simulink model "testUDPReceiveRoute"  (R2024a)
settings: Solver=FixedStepAuto  StartTime=0.0  StopTime=inf  FixedStep=1e-3  RelTol=1e-3
model workspace (MAT data in the model file):
  teste = Simulink.Parameter
  teste.Value = "Variable1"
  teste.Complexity = 'real'
  teste.Dimensions = [1 1]
  teste.DataType = 'string'
  teste1 = Simulink.Parameter
  teste1.Value = 1
  teste1.Complexity = 'real'
  teste1.Dimensions = [1 1]
  teste1.DataType = 'auto'
libraries: slrealtimeutilitieslib x1, slrealtimetgmanagement x1, slrealtimeiplib x1
settings Model: Creator=matlab.cut  LastModifiedBy=matlab.cut
settings SolverCC: ConcurrentTasks=on  PositivePriorityOrder=on
settings OptimizationCC: BlockReduction=off  OptimizeBlockIOStorage=off
settings DebuggingCC: TasksWithSamePriorityMsg=none
settings HardwareCC: ProdBitPerLong=64  ProdLongLongMode=on  ProdHWDeviceType=Intel->x86-64 (Linux 64)
settings RTWCC: Description=Speedgoat Real-Time Target Machine  SystemTargetFile=speedgoat.tlc  TemplateMakefile=slrealtime_default_tmf  Toolchain=Simulink Real-Time Toolchain  BuildConfiguration=Faster Runs  CodeExecutionProfiling=on  TargetLang=C++
settings SimulinkRealTimeTargetCC: InstructionSetFMA=off  LogToMDFFile=off

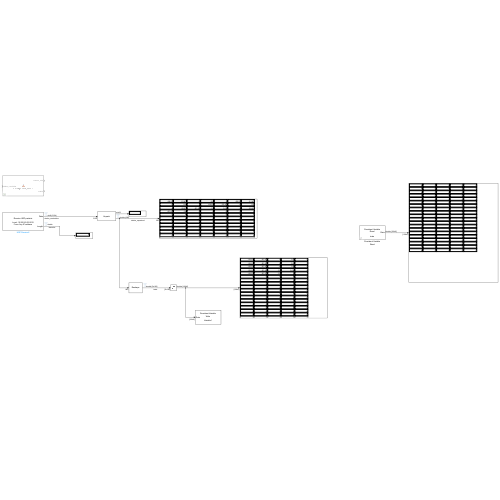
[thumbnail: Simulink's stored preview of the top-level diagram]
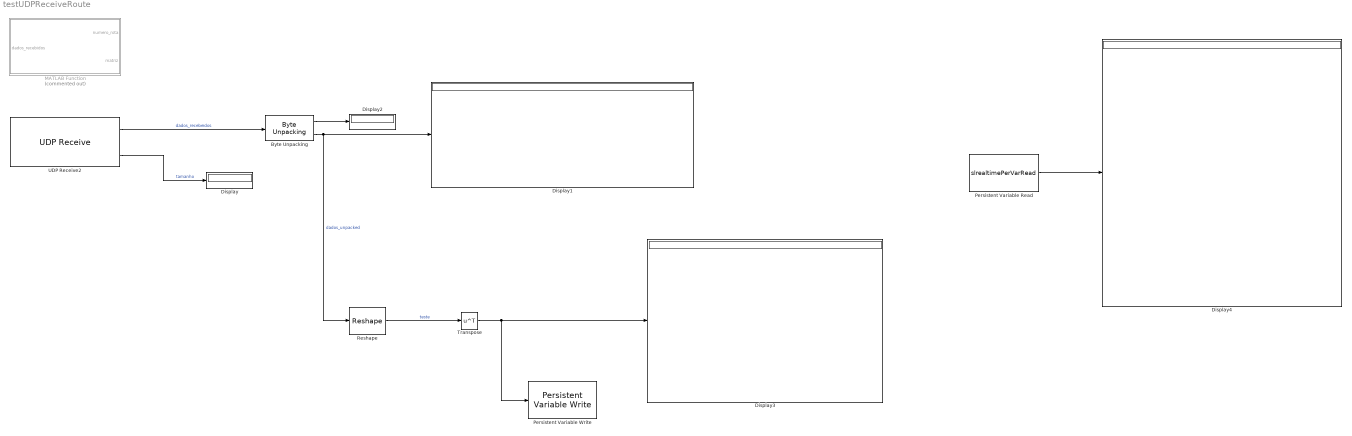
== system testUDPReceiveRoute ==
  Byte Unpacking : slrealtimeutilitieslib/Byte Unpacking  MaskUnpackedDataTypes={'uint32','double'}  MaskUnpackedDataSizes={[1],[640]}  MaskAlignment=1
  Display{,1..4} (5 alike) : Display
  MATLAB Function : MATLAB Function  Commented=on  TreatAsAtomicUnit=on
  Persistent Variable Read : S-Function  AncestorBlock=slrealtimetgmanagement/Persistent Variable Read  FunctionName=slrealtimePerVarRead  Parameters=varName defaultValue  SFunctionDeploymentMode=off  EnableBusSupport=off  mask(slrealtimepervarread){varName=teste, defaultValue=zeros(128, 5)}
      mask prompts: varName "slrealtime:persistentVar:variableName"; defaultValue "slrealtime:persistentVar:defaultValue"
      mask help: slrealtime:persistentVar:perVarReadDescription
      mask Help: eval('slrealtimedoc(''persistent_variable_read'')');
      mask Callback varName: slrealtime.internal.tgmgmt.PerVarRead.varNameCheck(gcb);
      mask DialogControl DescGroupVar Prompt: Persistent Variable Read
      mask DialogControl varName Prompt: Variable name
      mask DialogControl defaultValue Prompt: Default value
      mask Display:
      | if bdIsLibrary(bdroot)
      |     dispStr = getString(message('slrealtime:persistentVar:perVarReadDisp'));
      | else
      |     dispStr = [getString(message('slrealtime:persistentVar:perVarReadDisp')), ...
      |                '\n\n', ...
      |                get_param(gcb, 'varName')];
      | end
      | disp(dispStr);
      | 
      | port_label('output', 1, getString(message('slrealtime:persistentVar:data')));
  Persistent Variable Write : slrealtimetgmanagement/Persistent Variable Write  varName=Variable1
  Reshape : Reshape  OutputDimensionality=Customize  OutputDimensions=[5,128]
  Transpose : Math  Operator=transpose
  UDP Receive2 : slrealtimeiplib/UDP Receive  useHostTargetConn=off  ipAddress=10.200.83.53  localPort=5015  rcvWidth=5124  rcvFmAny=on  fmAddress='10.200.83.57'  sampleTime=1  enableMessage=off  maxPackets=1
  wires:
  UDP Receive2/1 -> Byte Unpacking/1  "dados_recebeidos"
  UDP Receive2/2 -> Display/1  "tamanho"
  Byte Unpacking/2 -> Display1/1, Reshape/1  "dados_unpacked"
  Reshape/1 -> Transpose/1  "teste"
  Transpose/1 -> Persistent Variable Write/1, Display3/1
  Persistent Variable Read/1 -> Display4/1
  Byte Unpacking/1 -> Display2/1

== matlab function testUDPReceiveRoute/MATLAB Function ==
  data: dados_recebidos input size=65507; numero_rota output; matriz output
function [numero_rota, matriz] = desempacotar_dados(dados_recebidos)
  
    % Número de bytes para o número da rota (int32 - 4 bytes)
    tamanho_numero_rota = 4;

    % Extrair o número da rota (int32 - 4 bytes)
    numero_rota = typecast(dados_recebidos(1:tamanho_numero_rota), 'int32');
    
    % Extrair os dados restantes e converter para matriz
    dados_resto = typecast(dados_recebidos(tamanho_numero_rota + 1:end), 'double');
    
    % Reformular os dados para uma matriz
    matriz = reshape(dados_resto, [], 5);
end
